simulink model "FullyActHexarotor"  (R2024b)
settings: Solver=ode3  StartTime=0.0  StopTime=100000  FixedStep=basic_step_time  RelTol=1e-3
values from neighbouring files (symbols this model uses):
  F = [F1; F2]    [design_param_optimization.m]
  g = 9.81    [design_param_optimization.m]
  m = 2    [design_param_optimization.m]
undefined symbols (not defined in the file or in its folder): J, k_i_p, k_i_R, k_omega, k_p, k_R, k_v, omega_init, p_init, R_init, v_init
libraries: sharedtransform x3, dspnetwork x1
settings Model: Creator=RyllM  LastModifiedBy=tham
settings DebuggingCC: UnconnectedInputMsg=warning  UnconnectedOutputMsg=warning  UnconnectedLineMsg=warning  UnderSpecifiedDimensionMsg=warning
settings ModelReferenceCC: EnableRefExpFcnMdlSchedulingChecks=on
settings RTWCC: GPUComputeCapability=3.5  DLArmComputeVersion=19.05

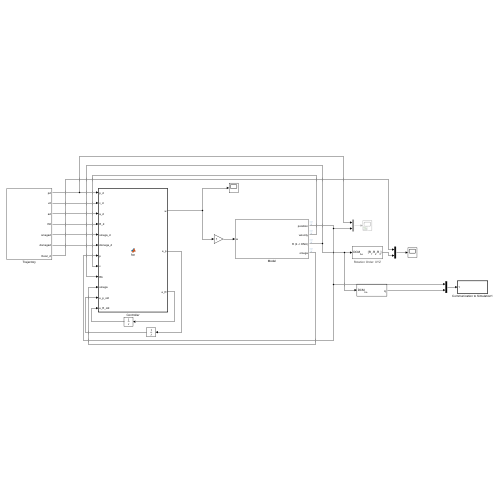
[thumbnail: Simulink's stored preview of the top-level diagram]
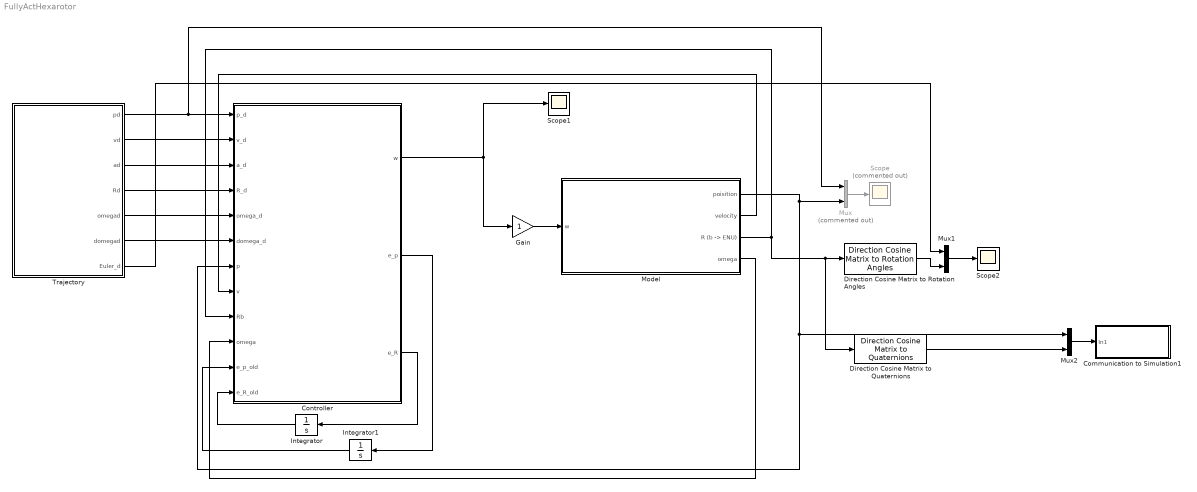
== system FullyActHexarotor ==
  Communication to Simulation1 : Subsystem  TreatAsAtomicUnit=on  SystemSampleTime=0.01
  Controller : MATLAB Function  TreatAsAtomicUnit=on
  Direction Cosine Matrix to Rotation Angles : sharedtransform/Direction Cosine Matrix to Rotation Angles  rotationOrder=XYZ  aMode=aMode  action=None  tolerance=eps(2)
  Direction Cosine Matrix to Quaternions : sharedtransform/Direction Cosine Matrix  to Quaternions  aMode=0  action=None  tolerance=eps(2)
  Gain : Gain
  Integrator : Integrator
  Integrator1 : Integrator
  Model : Subsystem
  Mux : Mux  Commented=on  Inputs=2
  Mux1 : Mux  Inputs=2
  Mux2 : Mux  Inputs=2
  Scope : Scope  Commented=on
  Scope1 : Scope
  Scope2 : Scope
  Trajectory : Subsystem
  wires:
  Controller/1(w) -> Scope1/1, Gain/1
  Trajectory/6(domegad) -> Controller/6(domega_d)
  Trajectory/5(omegad) -> Controller/5(omega_d)
  Trajectory/4(Rd) -> Controller/4(R_d)
  Trajectory/3(ad) -> Controller/3(a_d)
  Trajectory/2(vd) -> Controller/2(v_d)
  Trajectory/1(pd) -> Mux/1, Controller/1(p_d)
  Model/2(velocity) -> Controller/8(v)
  Model/4(omega) -> Controller/10(omega)
  Mux/1 -> Scope/1
  Mux1/1 -> Scope2/1
  Direction Cosine Matrix to Rotation Angles/1 -> Mux1/2
  Trajectory/7(Euler_d) -> Mux1/1
  Direction Cosine Matrix to Quaternions/1 -> Mux2/2
  Model/1(poisition) -> Controller/7(p), Mux2/1, Mux/2
  Mux2/1 -> Communication to Simulation1/1(In1)
  Model/3("R (b -> ENU)") -> Direction Cosine Matrix to Quaternions/1, Direction Cosine Matrix to Rotation Angles/1, Controller/9(Rb)
  Gain/1 -> Model/1(w)
  Controller/3(e_R) -> Integrator/1
  Integrator/1 -> Controller/12(e_R_old)
  Controller/2(e_p) -> Integrator1/1
  Integrator1/1 -> Controller/11(e_p_old)

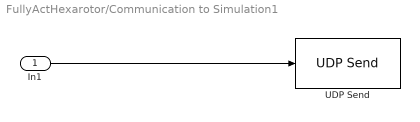
== system FullyActHexarotor/Communication to Simulation1 ==
  In1 : Inport
  UDP Send : dspnetwork/UDP Send  remoteURL='localhost'  remotePort=12346  localURL='0.0.0.0'  localPortSource=Automatically determine  localPort=-1  sendBufferSize=1  sampletime=-1  blockPlatform=[]  separateLengthPort=0
  wires:
  In1/1 -> UDP Send/1

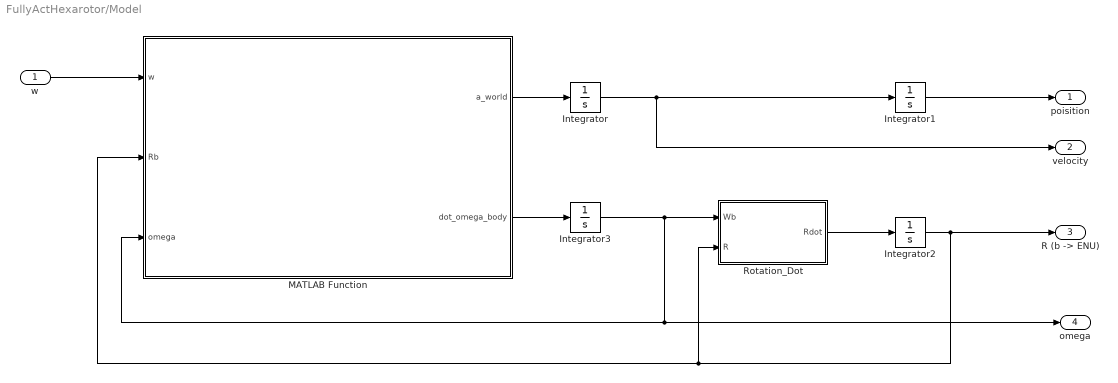
== system FullyActHexarotor/Model ==
  w : Inport
  Integrator : Integrator  InitialCondition=v_init
  Integrator1 : Integrator  InitialCondition=p_init
  Integrator2 : Integrator  InitialCondition=R_init
  Integrator3 : Integrator  InitialCondition=omega_init
  MATLAB Function : MATLAB Function  TreatAsAtomicUnit=on
  Rotation_Dot : MATLAB Function  TreatAsAtomicUnit=on
  poisition : Outport
  velocity : Outport  Port=2
  "R (b -> ENU)" : Outport  Port=3
  omega : Outport  Port=4
  wires:
  Integrator/1 -> velocity/1, Integrator1/1
  Integrator2/1 -> "R (b -> ENU)"/1, MATLAB Function/2(Rb), Rotation_Dot/2(R)
  Integrator1/1 -> poisition/1
  Integrator3/1 -> MATLAB Function/3(omega), omega/1, Rotation_Dot/1(Wb)
  Rotation_Dot/1(Rdot) -> Integrator2/1
  w/1 -> MATLAB Function/1(w)
  MATLAB Function/2(dot_omega_body) -> Integrator3/1
  MATLAB Function/1(a_world) -> Integrator/1

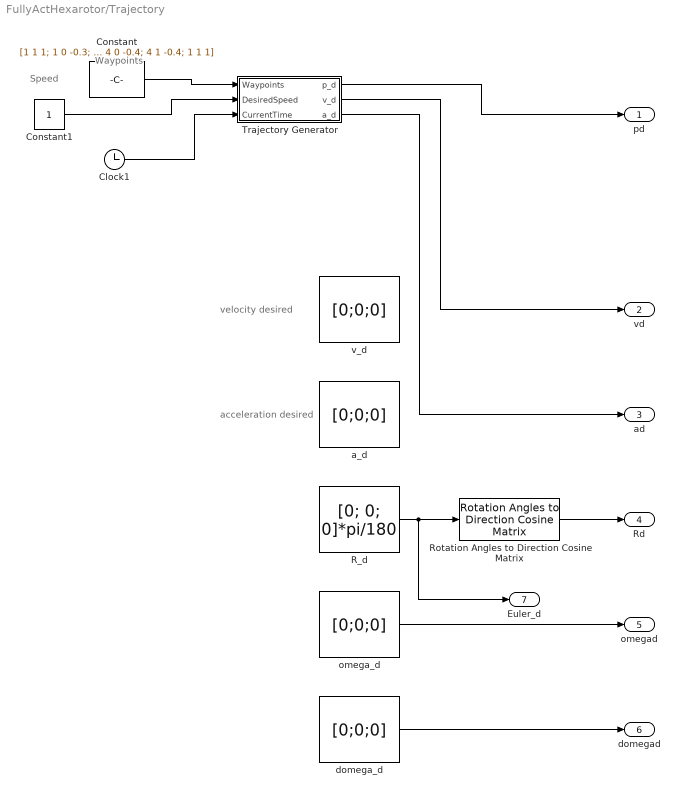
== system FullyActHexarotor/Trajectory ==
  note: Waypoints
  note: velocity desired
  note: acceleration desired
  note: Speed
  Clock1 : Clock
  Constant : Constant  Value=[1 1 1; 1 0 -0.3; 1 0.5 -0.4; 1 0 -0.4; 1 0 1; 4 0 1; 4 0 -0.4; 4 1 -0.4; 1 1 1]  VectorParams1D=off
  Constant1 : Constant
  R_d : Constant  Value=[0; 0; 0]*pi/180
  Rotation Angles to Direction Cosine Matrix : sharedtransform/Rotation Angles to Direction Cosine Matrix  rotationOrder=XYZ  aMode=aMode
  Trajectory Generator : Subsystem
  a_d : Constant  Value=[0;0;0]
  domega_d : Constant  Value=[0;0;0]
  omega_d : Constant  Value=[0;0;0]
  v_d : Constant  Value=[0;0;0]
  pd : Outport
  vd : Outport  Port=2
  ad : Outport  Port=3
  Rd : Outport  Port=4
  omegad : Outport  Port=5
  domegad : Outport  Port=6
  Euler_d : Outport  Port=7
  wires:
  R_d/1 -> Euler_d/1, Rotation Angles to Direction Cosine Matrix/1
  omega_d/1 -> omegad/1
  domega_d/1 -> domegad/1
  Rotation Angles to Direction Cosine Matrix/1 -> Rd/1
  Trajectory Generator/1(p_d) -> pd/1
  Constant/1 -> Trajectory Generator/1(Waypoints)
  Clock1/1 -> Trajectory Generator/3(CurrentTime)
  Constant1/1 -> Trajectory Generator/2(DesiredSpeed)
  Trajectory Generator/2(v_d) -> vd/1
  Trajectory Generator/3(a_d) -> ad/1

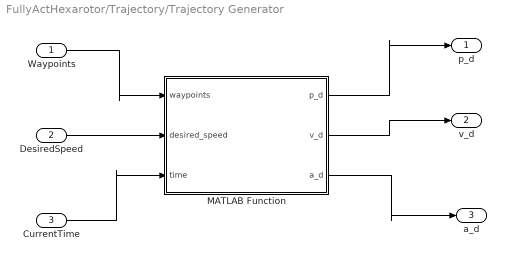
== system FullyActHexarotor/Trajectory/Trajectory Generator ==
  Waypoints : Inport
  DesiredSpeed : Inport  Port=2
  CurrentTime : Inport  Port=3
  MATLAB Function : MATLAB Function  TreatAsAtomicUnit=on
  p_d : Outport
  v_d : Outport  Port=2
  a_d : Outport  Port=3
  wires:
  Waypoints/1 -> MATLAB Function/1(waypoints)
  DesiredSpeed/1 -> MATLAB Function/2(desired_speed)
  CurrentTime/1 -> MATLAB Function/3(time)
  MATLAB Function/1(p_d) -> p_d/1
  MATLAB Function/2(v_d) -> v_d/1
  MATLAB Function/3(a_d) -> a_d/1

== matlab function FullyActHexarotor/Controller ==
  data: p_d input; w output; v_d input; a_d input; R_d input; omega_d input; domega_d input; p input; v input; Rb input; omega input; k_p parameter; k_v parameter; k_R parameter; k_omega parameter; m parameter; J parameter; F parameter; g parameter; e_p_old input; e_R_old input; e_p output; e_R output; k_i_p parameter; k_i_R parameter
function [w, e_p, e_R] = fcn(p_d, v_d, a_d, R_d, omega_d, domega_d, p, v, Rb, omega, k_p, k_v, k_R, k_omega, m, J, F, g, e_p_old, e_R_old, k_i_p, k_i_R)
    % k_v, k_p, k_i_p,  k_omega, k_R, k_i_R controller gains
    % Rb = R
    e_v = v - v_d;
    e_p = p - p_d;

    e_w = omega - Rb' * R_d * omega_d;
    e_R = 0.5 * unskew(R_d' * Rb - Rb' * R_d);
    

    v_p = a_d - k_v * e_v - k_p * e_p - k_i_p * e_p_old;
    v_r = domega_d - k_omega * e_w - k_R * e_R - k_i_R * e_R_old;
%     assignin('base', 'v_p_simulink', v_p);
% assignin('base', 'v_r_simulink', v_r);
% assignin('base', 'u_simulink', u);
%     fprintf('\n', size(v_p,1), size(v_p,2));
%     fprintf('\n', size(v_r,1), size(v_r,2));
%     v_r = reshape(v_r, [], 1);  % Convert to column vector if needed
%     v_p = reshape(v_p, [], 1);  % Convert to column vector if needed
    
    v = [v_p; v_r'];
    combined_v  = reshape(v, [6, 1]);
    %v = zeros(6, 1);  % Define w as a 6x1 column vector

    % Create matrices for dynamics
    zero = zeros(3, 3);
    mass = m * eye(3, 3);
    Jacobian = [Rb, zero; zero, eye(3)] * F;
    f = [0; 0; -m * g; cross(omega, J * omega)];
    
    % Calculate control input
    u = inv(Jacobian) * (- f + [mass, zero; zero, J] * combined_v);
    w = zeros(6, 1, 'double');


    % Calculate motor commands with explicit reshape
    w = sign(u) .* sqrt(abs(u));
    w = reshape(w, [6, 1]);

    
function res=unskew(u)

    res=[u(3,2);
        u(1,3);
        u(2,1)];
end
end

== matlab function FullyActHexarotor/Model/MATLAB Function ==
  data: w input; a_world output size=[3; 1]; dot_omega_body output; Rb input; F parameter; m parameter; J parameter; g parameter; omega input
function [a_world,dot_omega_body] = fcn(w, Rb, F, m, J, g, omega)
    % Rb = R
    u = sign(w) .* w.^2;
    a_world = [0 0 0]';
    dot_omega_body = [0 0 0]';
    
    zero = zeros(3, 3);
    mass = [1/m, 0, 0;
            0, 1/m, 0;
            0, 0, 1/m;];
    
    Jacobian = [mass, zero; zero, inv(J)] * [Rb, zero; zero, eye(3)] * F;
    f = [0; 0; -g; inv(J) * cross(omega, J * omega)];
    
    state = f + (Jacobian * u);
    
    a_world = state(1:3,1);
    dot_omega_body = state(4:6,1);

== matlab function FullyActHexarotor/Model/Rotation_Dot ==
  settings: updateMethod=DISCRETE
  data: Wb input; R input; Rdot output
function Rdot = Rototation_Dot(Wb,R)

p = Wb(1);
q = Wb(2);
r = Wb(3);

persistent Ro;

if isempty(Ro)
    Ro=[1   0   0;
        0   1   0;
        0   0   1];
else
    Ro= R;
end

Rdot= skew(p,q,r)*Ro;

function res=skew(p,q,r)

res=[0 -r q;
    r 0 -p;
    -q p 0];

== matlab function FullyActHexarotor/Trajectory/Trajectory Generator/MATLAB Function ==
  data: waypoints input; p_d output; desired_speed input; time input; v_d output; a_d output
function [p_d, v_d, a_d] = fcn(waypoints, desired_speed, time)
    % Wrapper function that computes desired position, velocity, and acceleration
    % for a given trajectory defined by waypoints and desired speed at a specific time.
    [p_d, v_d, a_d] = trajectory_generator(waypoints, desired_speed, time);
end

function [p_d, v_d, a_d] = trajectory_generator(waypoints, desired_speed, time)
    % Main function for generating a smooth trajectory based on waypoints.
    % It computes segment times, velocities, polynomial coefficients, and
    % evaluates the trajectory at a given time.

    segment_times = calculate_segment_times(waypoints, desired_speed);  % Determine time allocated for each segment
    velocities = compute_waypoint_velocities(waypoints);                % Estimate direction of motion at each waypoint
    velocities = velocities * desired_speed;                            % Scale unit directions by desired speed
    accelerations = zeros(size(waypoints));                             % Assume zero acceleration at waypoints

    % Get polynomial coefficients for trajectory segments
    coeffs = generate_polynomial_coefficients(waypoints, velocities, accelerations, segment_times);

    % Identify which segment the current time falls into
    [segment_idx, local_time] = find_current_segment(time, segment_times);

    % Evaluate trajectory (position, velocity, acceleration) at this moment
    [p_d, v_d, a_d] = evaluate_trajectory(coeffs, segment_idx, local_time);
end

function segment_times = calculate_segment_times(waypoints, desired_speed)
    % Computes cumulative segment times between waypoints based on distance and speed.

    n = size(waypoints, 1);
    segment_times = zeros(n, 1);  % Initialize time vector

    for i = 2:n
        segment_length = norm(waypoints(i,:) - waypoints(i-1,:));
        segment_times(i) = segment_times(i-1) + max(segment_length / desired_speed, 0.1);  % Avoid zero-time segments
    end
end

function velocities = compute_waypoint_velocities(waypoints)
    % Estimates the direction of travel at each waypoint using a bisector-based smoothing method.

    n = size(waypoints, 1);
    velocities = zeros(size(waypoints));

    % First waypoint: look towards the next waypoint
    if n > 1
        direction = waypoints(2,:) - waypoints(1,:);
        velocities(1,:) = direction / norm(direction);
    end

    % Intermediate waypoints: compute smoothed direction using bisectors
    for i = 2:n-1
        v_in = waypoints(i,:) - waypoints(i-1,:);
        v_out = waypoints(i+1,:) - waypoints(i,:);

        v_in_norm = v_in / norm(v_in);
        v_out_norm = v_out / norm(v_out);

        bisector = v_in_norm + v_out_norm;

        % Normalize and scale based on half angle between segments
        bisector = bisector / norm(bisector);
        cos_angle = dot(v_in_norm, v_out_norm);
        angle = acos(max(min(cos_angle, 1), -1));  % Clamp to avoid NaN from acos

        scale_factor = cos(angle/2);  % Smaller angles result in higher speeds
        velocities(i,:) = bisector * scale_factor;
    end

    % Last waypoint: look back toward the previous waypoint
    if n > 1
        direction = waypoints(n,:) - waypoints(n-1,:);
        velocities(n,:) = direction / norm(direction);
    end
end

function coeffs = generate_polynomial_coefficients(waypoints, velocities, accelerations, segment_times)
    % Computes the coefficients of 5th-degree polynomials for each segment
    % based on boundary conditions for position, velocity, and acceleration.

    n = size(waypoints, 1) - 1;
    coeffs.x = zeros(n, 6);
    coeffs.y = zeros(n, 6);
    coeffs.z = zeros(n, 6);

    for i = 1:n
        t0 = segment_times(i);
        t1 = segment_times(i+1);

        p0 = waypoints(i,:);
        p1 = waypoints(i+1,:);
        v0 = velocities(i,:);
        v1 = velocities(i+1,:);
        a0 = accelerations(i,:);
        a1 = accelerations(i+1,:);

        for dim = 1:3
            % Construct the system of equations for 5th-degree polynomial
            A = [1, t0, t0^2, t0^3, t0^4, t0^5;
                 0, 1, 2*t0, 3*t0^2, 4*t0^3, 5*t0^4;
                 0, 0, 2, 6*t0, 12*t0^2, 20*t0^3;
                 1, t1, t1^2, t1^3, t1^4, t1^5;
                 0, 1, 2*t1, 3*t1^2, 4*t1^3, 5*t1^4;
                 0, 0, 2, 6*t1, 12*t1^2, 20*t1^3];

            b = [p0(dim); v0(dim); a0(dim); p1(dim); v1(dim); a1(dim)];
            c = A \ b;  % Solve linear system for coefficients

            % Store coefficients by dimension
            switch dim
                case 1, coeffs.x(i,:) = c';
                case 2, coeffs.y(i,:) = c';
                case 3, coeffs.z(i,:) = c';
            end
        end
    end
end

function [segment_idx, local_time] = find_current_segment(time, segment_times)
    % Determines which segment the current time falls into,
    % and returns the local time within that segment.

    n = length(segment_times) - 1;
    segment_idx = n;
    local_time = time;

    for i = 1:n
        if time >= segment_times(i) && time < segment_times(i+1)
            segment_idx = i;
            local_time = time;
            return;
        end
    end

    % Clamp to final segment if time is beyond final waypoint
    if time >= segment_times(end)
        segment_idx = n;
        local_time = segment_times(end);
    end
end

function [pos, vel, acc] = evaluate_trajectory(coeffs, segment_idx, t)
    % Evaluates the polynomial trajectory at time t within a specific segment,
    % returning position, velocity, and acceleration.

    cx = coeffs.x(segment_idx,:);
    cy = coeffs.y(segment_idx,:);
    cz = coeffs.z(segment_idx,:);

    % Position
    pos = [polyval(flip(cx), t), polyval(flip(cy), t), polyval(flip(cz), t)];

    % Velocity: first derivative
    vel = [polyval(polyder(flip(cx)), t), ...
           polyval(polyder(flip(cy)), t), ...
           polyval(polyder(flip(cz)), t)];

    % Acceleration: second derivative
    acc = [polyval(polyder(polyder(flip(cx))), t), ...
           polyval(polyder(polyder(flip(cy))), t), ...
           polyval(polyder(polyder(flip(cz))), t)];
end
